simulink model "lab_1"  (R2016a)
settings: Solver=VariableStepAuto  SolverMode=SingleTasking  StartTime=0.0  StopTime=10  RelTol=1e-3
settings Model: Creator=Универская хуета  LastModifiedBy=Универская хуета
settings DataIOCC: LimitDataPoints=on  SaveOutput=off  SaveTime=off
settings OptimizationCC: BlockReduction=off  BooleanDataType=off
settings DebuggingCC: SaveWithParameterizedLinksMsg=none  UnderspecifiedInitializationDetection=Classic  MergeDetectMultiDrivingBlocksExec=none  SignalResolutionControl=TryResolveAllWithWarning  AllowSymbolicDim=off
settings HardwareCC: TargetUnknown=on

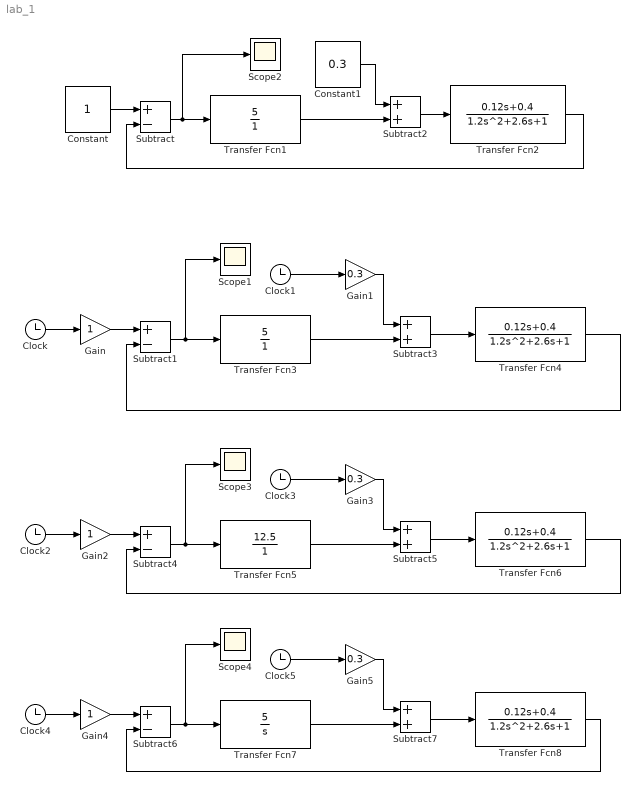
== system lab_1 ==
  Clock{,1..5} (6 alike) : Clock
  Constant : Constant
  Constant1 : Constant  Value=0.3
  Gain : Gain
  Gain1 : Gain  Gain=0.3
  Gain2 : Gain
  Gain3 : Gain  Gain=0.3
  Gain4 : Gain
  Gain5 : Gain  Gain=0.3
  Scope{1..4} (4 alike) : Scope
  Subtract{,1,4,6} (4 alike) : Sum  Inputs=+-
  Subtract{2..3,5,7} (4 alike) : Sum
  Transfer Fcn1 : TransferFcn  Numerator=[5]  Denominator=[1]
  Transfer Fcn{2,4,6,8} (4 alike) : TransferFcn  Numerator=[0.12 0.4]  Denominator=[1.2 2.6 1]
  Transfer Fcn3 : TransferFcn  Numerator=[5]  Denominator=[1]
  Transfer Fcn5 : TransferFcn  Numerator=[12.5]  Denominator=[1]
  Transfer Fcn7 : TransferFcn  Numerator=5  Denominator=[1 0]
  wires:
  Constant/1 -> Subtract/1
  Transfer Fcn1/1 -> Subtract2/2
  Transfer Fcn2/1 -> Subtract/2
  Constant1/1 -> Subtract2/1
  Subtract/1 -> Transfer Fcn1/1, Scope2/1
  Transfer Fcn3/1 -> Subtract3/2
  Transfer Fcn4/1 -> Subtract1/2
  Subtract1/1 -> Transfer Fcn3/1, Scope1/1
  Gain/1 -> Subtract1/1
  Clock/1 -> Gain/1
  Clock1/1 -> Gain1/1
  Gain1/1 -> Subtract3/1
  Subtract2/1 -> Transfer Fcn2/1
  Subtract3/1 -> Transfer Fcn4/1
  Transfer Fcn5/1 -> Subtract5/2
  Transfer Fcn6/1 -> Subtract4/2
  Subtract4/1 -> Transfer Fcn5/1, Scope3/1
  Gain2/1 -> Subtract4/1
  Clock2/1 -> Gain2/1
  Clock3/1 -> Gain3/1
  Gain3/1 -> Subtract5/1
  Subtract5/1 -> Transfer Fcn6/1
  Transfer Fcn7/1 -> Subtract7/2
  Transfer Fcn8/1 -> Subtract6/2
  Subtract6/1 -> Transfer Fcn7/1, Scope4/1
  Gain4/1 -> Subtract6/1
  Clock4/1 -> Gain4/1
  Clock5/1 -> Gain5/1
  Gain5/1 -> Subtract7/1
  Subtract7/1 -> Transfer Fcn8/1
